simulink model "pid_with_sfun"  (R2019a)
settings: Solver=ode8  StartTime=tspan(1)  StopTime=tspan(end)  FixedStep=0.05  RelTol=1e-3
values from neighbouring files (symbols this model uses):
  fin_step = -25    [pid_with_simulink.m]
  fin_steptime = 25    [pid_with_simulink.m]
  fout_max = 2*fss    (= 600)    [pid_with_simulink.m]
  fout_min = 0    [pid_with_simulink.m]
  fss = 300    [pid_with_simulink.m]
  kc1 = -2    [pid_with_simulink.m]
  kc2 = 1e6    (= 1000000)    [pid_with_simulink.m]
  q_max = 2*qss    (= 100464000)    [pid_with_simulink.m]
  q_min = 0    [pid_with_simulink.m]
  qss = fss*RHO*CP*(tss-tinss)    (= 50232000)    [pid_with_simulink.m]
  ti2 = 0.5    [pid_with_simulink.m]
  tin_step = 0    [pid_with_simulink.m]
  tin_steptime = 1    [pid_with_simulink.m]
  tinss = 30    [pid_with_simulink.m]
  tsp_step1 = 5    [pid_with_simulink.m]
  tsp_step2 = -10    [pid_with_simulink.m]
  tsp_steptime1 = 1    [pid_with_simulink.m]
  tsp_steptime2 = 12    [pid_with_simulink.m]
  tss = 70    [pid_with_simulink.m]
  vss = vmax/2    (= 100)    [pid_with_simulink.m]
libraries: simulink x2
settings Model: Creator=Mike  LastModifiedBy=Mike
settings DataIOCC: ReturnWorkspaceOutputs=off

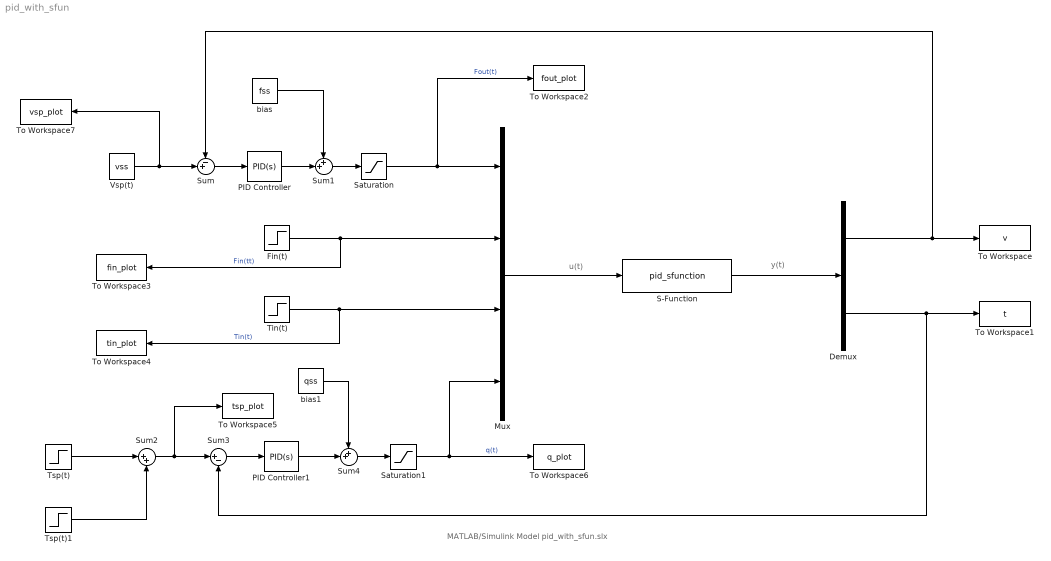
== system pid_with_sfun ==
  note: u(t)
  note: MATLAB/Simulink Model pid_with_sfun.slx
  note: y(t)
  Demux : Demux  Outputs=2
  Fin(t) : Step  Time=fin_steptime  Before=fss  After=fss+fin_step  SampleTime=0
  Mux : Mux
  PID Controller : simulink/Continuous/PID Controller  Controller=PID  Form=Parallel  TimeDomain=Continuous-time  SampleTime=-1  IntegratorMethod=Forward Euler  FilterMethod=Forward Euler  ControllerParametersSource=internal  P=kc1  I=0  D=0  UseFilter=on  N=100  TunerSelectOption=Transfer Function Based (PID Tuner App)  InitialConditionSource=internal  InitialConditionForIntegrator=0  InitialConditionForFilter=0  DifferentiatorICPrevScaledInput=0  ExternalReset=none  TrackingMode=off  Kt=1  LimitOutput=off  UpperSaturationLimit=fout_max  LowerSaturationLimit=fout_min  LinearizeAsGain=on  AntiWindupMode=none  Kb=1  POutMin=[]  POutMax=[]  IOutMin=[]  IOutMax=[]  DOutMin=[]  DOutMax=[]  NOutMin=[]  NOutMax=[]  SumOutMin=[]  SumOutMax=[]  SaturationOutMin=[]  SaturationOutMax=[]  PParamMin=[]  PParamMax=[]  IParamMin=[]  IParamMax=[]  DParamMin=[]  DParamMax=[]  NParamMin=[]  NParamMax=[]  KbParamMin=[]  KbParamMax=[]  KtParamMin=[]  KtParamMax=[]  KbOutMin=[]  KbOutMax=[]  KtOutMin=[]  KtOutMax=[]  IntegratorOutMin=[]  IntegratorOutMax=[]  FilterOutMin=[]  FilterOutMax=[]  SumI1OutMin=[]  SumI1OutMax=[]  SumI2OutMin=[]  SumI2OutMax=[]  SumI3OutMin=[]  SumI3OutMax=[]  SumI4OutMin=[]  SumI4OutMax=[]  SumDOutMin=[]  SumDOutMax=[]  DifferentiatorOutMin=[]  DifferentiatorOutMax=[]  FilterDiffOutCoefMin=[]  FilterDiffOutCoefMax=[]  ReciprocalOutMin=[]  ReciprocalOutMax=[]  SumDenOutMin=[]  SumDenOutMax=[]  SumNumOutMin=[]  SumNumOutMax=[]  DivideOutMin=[]  DivideOutMax=[]  IntegratorContinuousStateAttributes=''  IntegratorStateMustResolveToSignalObject=off  IntegratorRTWStateStorageClass=Auto  FilterContinuousStateAttributes=''  FilterStateMustResolveToSignalObject=off  FilterRTWStateStorageClass=Auto  ParallelPVariant=InternalParameters  IdealPVariant=Disabled  IVariant=InternalParameters  DVariant=InternalParameters  IntegratorVariant=Continuous  SatVariant=Disabled  AWVariant=Passthrough  PCopyVariant=Disabled  TRVariant=Disabled  FdbkBlocksVariant=Forward  IdealPFdbkVariant=Disabled  SatFdbkVariant=Disabled  DerivativeFilterVariant=ContFilter  NVariant=InternalParameters  NCopyVariant=Disabled  FilterICVariant=InternalICsFilter  IntegratorICVariant=InternalICs  ExternalResetVariant=Disabled  TRSumVariant=Passthrough  SumFdbkVariant=Disabled  SumVariant=Sum_PID
  PID Controller1 : simulink/Continuous/PID Controller  Controller=PID  Form=Parallel  TimeDomain=Continuous-time  SampleTime=-1  IntegratorMethod=Forward Euler  FilterMethod=Forward Euler  ControllerParametersSource=internal  P=kc2  I=kc2/ti2  D=0  UseFilter=on  N=100  TunerSelectOption=Transfer Function Based (PID Tuner App)  InitialConditionSource=internal  InitialConditionForIntegrator=0  InitialConditionForFilter=0  DifferentiatorICPrevScaledInput=0  ExternalReset=none  TrackingMode=off  Kt=1  LimitOutput=off  UpperSaturationLimit=q_max  LowerSaturationLimit=q_min  LinearizeAsGain=on  AntiWindupMode=none  Kb=1  POutMin=[]  POutMax=[]  IOutMin=[]  IOutMax=[]  DOutMin=[]  DOutMax=[]  NOutMin=[]  NOutMax=[]  SumOutMin=[]  SumOutMax=[]  SaturationOutMin=[]  SaturationOutMax=[]  PParamMin=[]  PParamMax=[]  IParamMin=[]  IParamMax=[]  DParamMin=[]  DParamMax=[]  NParamMin=[]  NParamMax=[]  KbParamMin=[]  KbParamMax=[]  KtParamMin=[]  KtParamMax=[]  KbOutMin=[]  KbOutMax=[]  KtOutMin=[]  KtOutMax=[]  IntegratorOutMin=[]  IntegratorOutMax=[]  FilterOutMin=[]  FilterOutMax=[]  SumI1OutMin=[]  SumI1OutMax=[]  SumI2OutMin=[]  SumI2OutMax=[]  SumI3OutMin=[]  SumI3OutMax=[]  SumI4OutMin=[]  SumI4OutMax=[]  SumDOutMin=[]  SumDOutMax=[]  DifferentiatorOutMin=[]  DifferentiatorOutMax=[]  FilterDiffOutCoefMin=[]  FilterDiffOutCoefMax=[]  ReciprocalOutMin=[]  ReciprocalOutMax=[]  SumDenOutMin=[]  SumDenOutMax=[]  SumNumOutMin=[]  SumNumOutMax=[]  DivideOutMin=[]  DivideOutMax=[]  IntegratorContinuousStateAttributes=''  IntegratorStateMustResolveToSignalObject=off  IntegratorRTWStateStorageClass=Auto  FilterContinuousStateAttributes=''  FilterStateMustResolveToSignalObject=off  FilterRTWStateStorageClass=Auto  ParallelPVariant=InternalParameters  IdealPVariant=Disabled  IVariant=InternalParameters  DVariant=InternalParameters  IntegratorVariant=Continuous  SatVariant=Disabled  AWVariant=Passthrough  PCopyVariant=Disabled  TRVariant=Disabled  FdbkBlocksVariant=Forward  IdealPFdbkVariant=Disabled  SatFdbkVariant=Disabled  DerivativeFilterVariant=ContFilter  NVariant=InternalParameters  NCopyVariant=Disabled  FilterICVariant=InternalICsFilter  IntegratorICVariant=InternalICs  ExternalResetVariant=Disabled  TRSumVariant=Passthrough  SumFdbkVariant=Disabled  SumVariant=Sum_PID
  S-Function : S-Function  FunctionName=pid_sfunction  SFunctionDeploymentMode=off  EnableBusSupport=off
  Saturation : Saturate  UpperLimit=fout_max  LowerLimit=fout_min
  Saturation1 : Saturate  UpperLimit=q_max  LowerLimit=q_min
  Sum : Sum  Inputs=-+|
  Sum1 : Sum  Inputs=++|
  Sum2 : Sum  Inputs=|++
  Sum3 : Sum  Inputs=|+-
  Sum4 : Sum  Inputs=++|
  Tin(t) : Step  Time=tin_steptime  Before=tinss  After=tinss+tin_step  SampleTime=0
  To Workspace : ToWorkspace  VariableName=v  SampleTime=-1
  To Workspace1 : ToWorkspace  VariableName=t  SampleTime=-1
  To Workspace2 : ToWorkspace  VariableName=fout_plot  SampleTime=-1
  To Workspace3 : ToWorkspace  VariableName=fin_plot  SampleTime=-1
  To Workspace4 : ToWorkspace  VariableName=tin_plot  SampleTime=-1
  To Workspace5 : ToWorkspace  VariableName=tsp_plot  SampleTime=-1
  To Workspace6 : ToWorkspace  VariableName=q_plot  SampleTime=-1
  To Workspace7 : ToWorkspace  VariableName=vsp_plot  SampleTime=-1
  Tsp(t) : Step  Time=tsp_steptime1  Before=tss  After=tss+tsp_step1  SampleTime=0
  Tsp(t)1 : Step  Time=tsp_steptime2  After=tsp_step2  SampleTime=0
  Vsp(t) : Constant  Value=vss
  bias : Constant  Value=fss
  bias1 : Constant  Value=qss
  wires:
  Mux/1 -> S-Function/1
  S-Function/1 -> Demux/1
  Demux/1 -> Sum/1, To Workspace/1
  Demux/2 -> To Workspace1/1, Sum3/2
  Vsp(t)/1 -> To Workspace7/1, Sum/2
  Sum/1 -> PID Controller/1
  PID Controller/1 -> Sum1/2
  bias/1 -> Sum1/1
  Fin(t)/1 -> To Workspace3/1, Mux/2  "Fin(tt)"
  Tin(t)/1 -> To Workspace4/1, Mux/3  "Tin(t)"
  Sum2/1 -> To Workspace5/1, Sum3/1
  Tsp(t)1/1 -> Sum2/2
  Tsp(t)/1 -> Sum2/1
  Sum3/1 -> PID Controller1/1
  PID Controller1/1 -> Sum4/2
  bias1/1 -> Sum4/1
  Sum1/1 -> Saturation/1
  Saturation/1 -> To Workspace2/1, Mux/1  "Fout(t)"
  Sum4/1 -> Saturation1/1
  Saturation1/1 -> Mux/4, To Workspace6/1  "q(t)"
